simulink model "punto1_taller_2"  (R2020b)
settings: Solver=VariableStepAuto  StartTime=0.0  StopTime=0.5  RelTol=1e-3
settings Model: Creator=User  LastModifiedBy=User

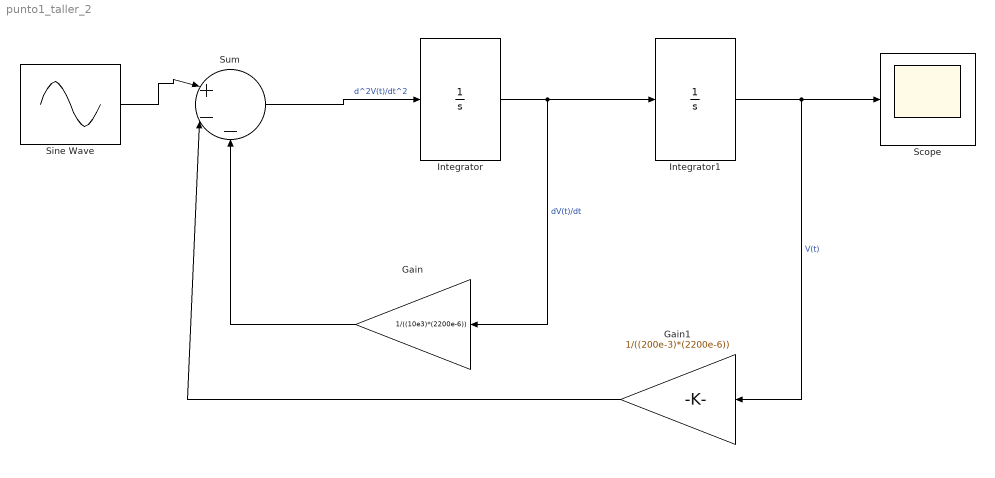
== system punto1_taller_2 ==
  Gain : Gain  Gain=1/((10e3)*(2200e-6))
  Gain1 : Gain  Gain=1/((200e-3)*(2200e-6))
  Integrator : Integrator
  Integrator1 : Integrator
  Scope : Scope
  Sine Wave : Sin  Amplitude=120  Frequency=2*pi*60  Phase=pi/2  SampleTime=0.00001
  Sum : Sum  Inputs=|+--
  wires:
  Integrator/1 -> Gain/1, Integrator1/1  "dV(t)/dt"
  Sum/1 -> Integrator/1  "d^2V(t)/dt^2"
  Gain/1 -> Sum/3
  Gain1/1 -> Sum/2
  Integrator1/1 -> Gain1/1, Scope/1  "V(t)"
  Sine Wave/1 -> Sum/1
